simulink library "crop_cost"  (R2025b)
settings: Solver=VariableStepAuto  StartTime=0.0  StopTime=10.0  RelTol=1e-3
settings Model: Creator=ciepm  LastModifiedBy=ciepm

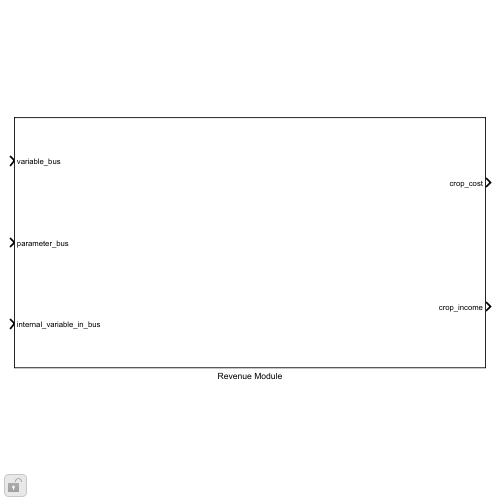
[thumbnail: Simulink's stored preview of the top-level diagram]
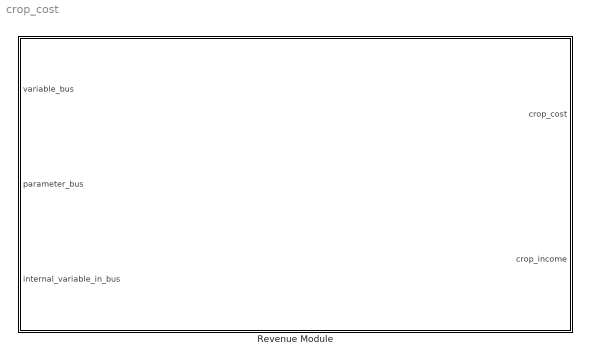
== system crop_cost ==
  Revenue Module : Subsystem

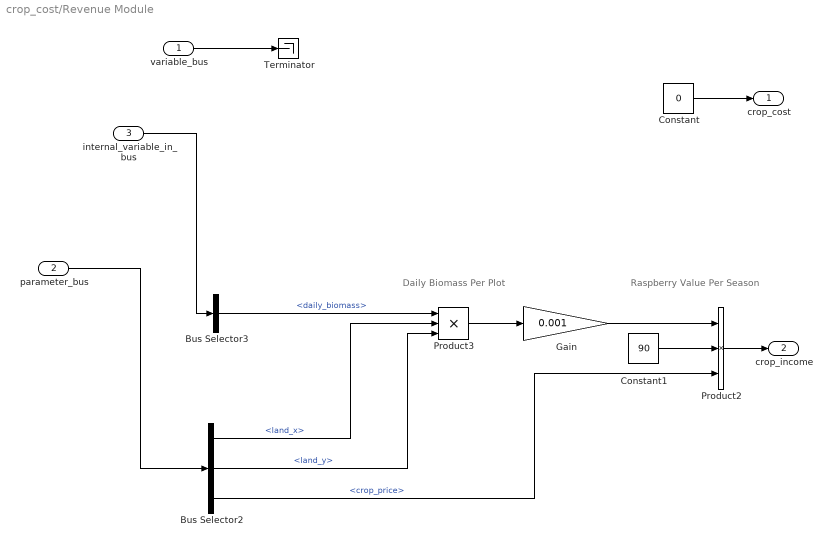
== system crop_cost/Revenue Module ==
  note: Daily Biomass Per Plot
  note: Raspberry Value Per Season
  variable_bus : Inport
  parameter_bus : Inport  Port=2
  internal_variable_in_bus : Inport  Port=3
  Bus Selector2 : BusSelector  OutputSignals=land_x,land_y,crop_price
  Bus Selector3 : BusSelector  OutputSignals=daily_biomass
  Constant : Constant  Value=0
  Constant1 : Constant  Value=90
  Gain : Gain  Gain=0.001
  Product2 : Product  Inputs=3
  Product3 : Product  Inputs=3
  Terminator : Terminator
  crop_cost : Outport
  crop_income : Outport  Port=2
  wires:
  Product2/1 -> crop_income/1
  Bus Selector3/1 -> Product3/1  "<daily_biomass>"
  Bus Selector2/1 -> Product3/2  "<land_x>"
  Bus Selector2/2 -> Product3/3  "<land_y>"
  Bus Selector2/3 -> Product2/3  "<crop_price>"
  Constant1/1 -> Product2/2
  Gain/1 -> Product2/1
  Product3/1 -> Gain/1
  Constant/1 -> crop_cost/1
  variable_bus/1 -> Terminator/1
  parameter_bus/1 -> Bus Selector2/1
  internal_variable_in_bus/1 -> Bus Selector3/1
